simulink model "DCmachine"  (R2023b)
settings: Solver=VariableStepAuto  StartTime=0.0  StopTime=30  RelTol=1e-3
values from neighbouring files (symbols this model uses):
  CM = 2.909*10^-5    (= 2.909e-05)    [dcdata.m]
  Ea = 12    [dcdata.m]
  Jm = 6.24*10^-4    (= 0.000624)    [dcdata.m]
  Kb = 1.7629*10^-2    (= 0.017629)    [dcdata.m]
  Kt = 1.7629*10^-2    (= 0.017629)    [dcdata.m]
  La = 0.28    [dcdata.m]
  Ra = 0.22680    (= 0.2268)    [dcdata.m]
  Trat = Ia*Kt    (= 0.158661)    [dcdata.m]
  wm = 564.9    [dcdata.m]
libraries: slpidlib x1
settings Model: Creator=helle  LastModifiedBy=helle

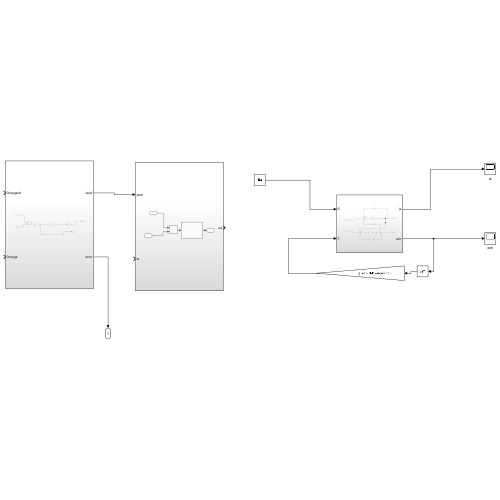
[thumbnail: Simulink's stored preview of the top-level diagram]
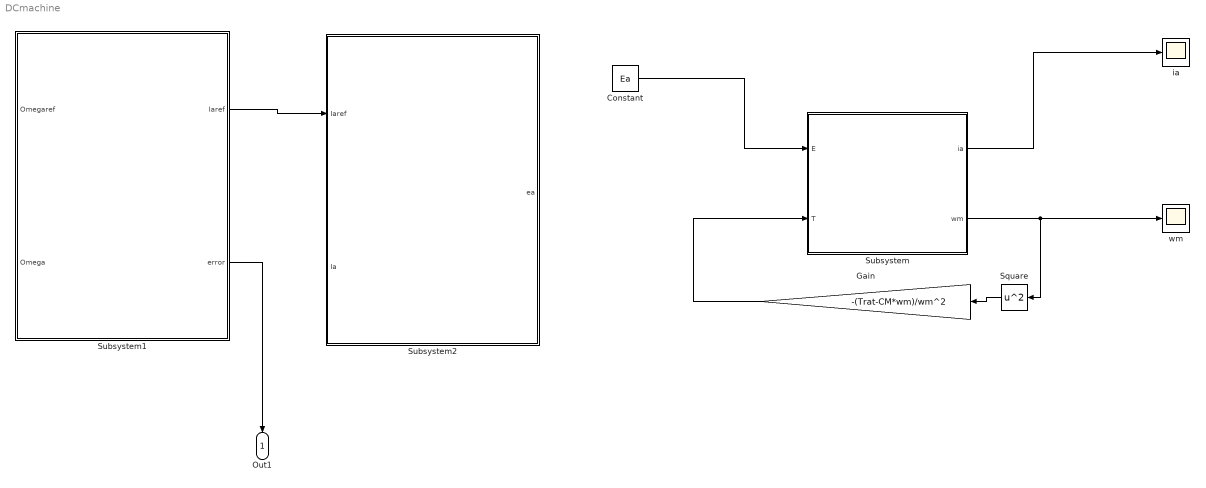
== system DCmachine ==
  Constant : Constant  Value=Ea
  Gain : Gain  Gain=-(Trat-CM*wm)/wm^2
  Square : Math  Operator=square
  Subsystem : Subsystem
  Subsystem1 : Subsystem
  Subsystem2 : Subsystem
  ia : Scope
  wm : Scope
  Out1 : Outport
  wires:
  Constant/1 -> Subsystem/1(E)
  Gain/1 -> Subsystem/2(T)
  Subsystem/1(ia) -> ia/1
  Subsystem/2(wm) -> Square/1, wm/1
  Square/1 -> Gain/1
  Subsystem1/1(Iaref) -> Subsystem2/1(Iaref)
  Subsystem1/2(error) -> Out1/1

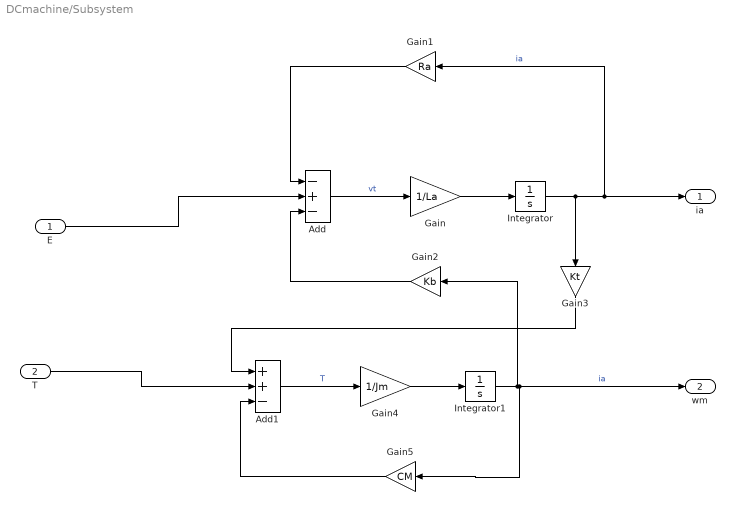
== system DCmachine/Subsystem ==
  E : Inport
  T : Inport  Port=2
  Add : Sum  Inputs=-+-
  Add1 : Sum  Inputs=++-
  Gain : Gain  Gain=1/La
  Gain1 : Gain  Gain=Ra
  Gain2 : Gain  Gain=Kb
  Gain3 : Gain  Gain=Kt
  Gain4 : Gain  Gain=1/Jm
  Gain5 : Gain  Gain=CM
  Integrator : Integrator
  Integrator1 : Integrator
  ia : Outport
  wm : Outport  Port=2
  wires:
  Gain2/1 -> Add/3
  Gain/1 -> Integrator/1
  Integrator1/1 -> Gain2/1, wm/1, Gain5/1  "ia"
  Add1/1 -> Gain4/1  "T"
  Add/1 -> Gain/1  "vt"
  Gain1/1 -> Add/1
  Gain4/1 -> Integrator1/1
  Integrator/1 -> ia/1, Gain1/1, Gain3/1  "ia"
  Gain3/1 -> Add1/1
  Gain5/1 -> Add1/3
  E/1 -> Add/2
  T/1 -> Add1/2

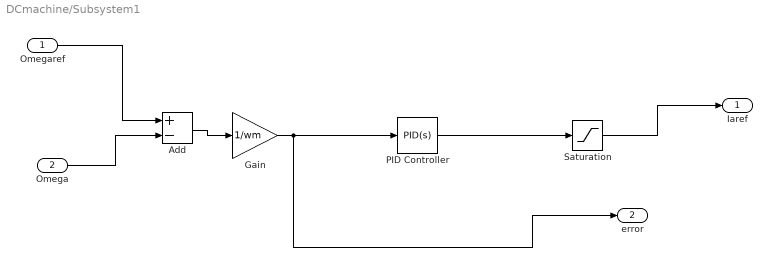
== system DCmachine/Subsystem1 ==
  Omegaref : Inport
  Omega : Inport  Port=2
  Add : Sum  Inputs=+-
  Gain : Gain  Gain=1/wm
  PID Controller : slpidlib/PID Controller  Controller=PID  Form=Parallel  TimeDomain=Continuous-time  UseExternalTs=off  SampleTime=-1  IntegratorMethod=Forward Euler  FilterMethod=Forward Euler  ControllerParametersSource=internal  P=1  I=1  UseKiTs=off  D=0  N=100  UseFilter=on  TunerSelectOption=Transfer Function Based (PID Tuner App)  InitialConditionSource=internal  InitialConditionForIntegrator=0  InitialConditionForFilter=0  DifferentiatorICPrevScaledInput=0  ExternalReset=none  TrackingMode=off  Kt=1  LimitOutput=off  SatLimitsSource=internal  UpperSaturationLimit=inf  LowerSaturationLimit=-inf  LinearizeAsGain=on  AntiWindupMode=none  Kb=1  LimitIntegrator=off  UpperIntegratorSaturationLimit=inf  LowerIntegratorSaturationLimit=-inf  POutMin=[]  POutMax=[]  IOutMin=[]  IOutMax=[]  DOutMin=[]  DOutMax=[]  NOutMin=[]  NOutMax=[]  SumOutMin=[]  SumOutMax=[]  SaturationOutMin=[]  SaturationOutMax=[]  PParamMin=[]  PParamMax=[]  IParamMin=[]  IParamMax=[]  DParamMin=[]  DParamMax=[]  NParamMin=[]  NParamMax=[]  KbParamMin=[]  KbParamMax=[]  KtParamMin=[]  KtParamMax=[]  KbOutMin=[]  KbOutMax=[]  KtOutMin=[]  KtOutMax=[]  IntegratorOutMin=[]  IntegratorOutMax=[]  FilterOutMin=[]  FilterOutMax=[]  SumI1OutMin=[]  SumI1OutMax=[]  SumI2OutMin=[]  SumI2OutMax=[]  SumI3OutMin=[]  SumI3OutMax=[]  SumI4OutMin=[]  SumI4OutMax=[]  SumDOutMin=[]  SumDOutMax=[]  DifferentiatorOutMin=[]  DifferentiatorOutMax=[]  FilterDiffOutCoefMin=[]  FilterDiffOutCoefMax=[]  ReciprocalOutMin=[]  ReciprocalOutMax=[]  SumDenOutMin=[]  SumDenOutMax=[]  SumNumOutMin=[]  SumNumOutMax=[]  DivideOutMin=[]  DivideOutMax=[]  UdiffTsProdOutMin=[]  UdiffTsProdOutMax=[]  NTsProdOutMin=[]  NTsProdOutMax=[]  UintegralTsProdOutMin=[]  UintegralTsProdOutMax=[]  UngainTsProdOutMin=[]  UngainTsProdOutMax=[]  ClampingZeroOutDataTypeStr=Inherit: Inherit via back propagation  ClampingZeroOutMin=[]  ClampingZeroOutMax=[]  FilterDenConstantOutDataTypeStr=Inherit: Inherit via back propagation  FilterDenConstantOutMin=[]  FilterDenConstantOutMax=[]  PCopyOutDataTypeStr=Inherit: Inherit via back propagation  PCopyOutMin=[]  PCopyOutMax=[]  NCopyOutDataTypeStr=Inherit: Inherit via back propagation  NCopyOutMin=[]  NCopyOutMax=[]  IntegratorContinuousStateAttributes=''  IntegratorStateMustResolveToSignalObject=off  IntegratorRTWStateStorageClass=Auto  FilterContinuousStateAttributes=''  FilterStateMustResolveToSignalObject=off  FilterRTWStateStorageClass=Auto  ParallelPVariant=InternalParameters  IdealPVariant=Disabled  IVariant=InternalParameters  DVariant=InternalParameters  IntegratorVariant=Continuous  SatVariant=Disabled  AWVariant=Passthrough  PCopyVariant=Disabled  TRVariant=Disabled  FdbkBlocksVariant=Forward  IdealPFdbkVariant=Disabled  SatFdbkVariant=Disabled  DerivativeFilterVariant=ContFilter  NVariant=InternalParameters  NCopyVariant=Disabled  FilterICVariant=InternalICsFilter  IntegratorICVariant=InternalICs  ExternalResetVariant=Disabled  TRSumVariant=Passthrough  SumFdbkVariant=Disabled  SumVariant=Sum_PID  TsampFilterVariant=InternalTs  TsampNgainVariant=Passthrough  TsampIntegralVariant=Passthrough  ExternalSaturationOutDataTypeStr=Inherit: Same as second input
  Saturation : Saturate
  Iaref : Outport
  error : Outport  Port=2
  wires:
  Omegaref/1 -> Add/1
  Omega/1 -> Add/2
  Add/1 -> Gain/1
  Gain/1 -> PID Controller/1, error/1
  Saturation/1 -> Iaref/1
  PID Controller/1 -> Saturation/1

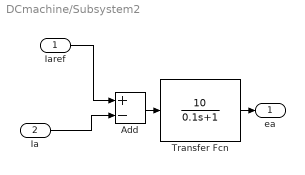
== system DCmachine/Subsystem2 ==
  Iaref : Inport
  Ia : Inport  Port=2
  Add : Sum  Inputs=+-
  Transfer Fcn : TransferFcn  Numerator=[10]  Denominator=[0.1 1]
  ea : Outport
  wires:
  Iaref/1 -> Add/1
  Ia/1 -> Add/2
  Add/1 -> Transfer Fcn/1
  Transfer Fcn/1 -> ea/1
